simulink model "roachf_2048ch"  (Simulink 7.5)
settings: Solver=ode45  StartTime=0.0  StopTime=10.0  RelTol=1e-3
undefined symbols (not defined in the file or in its folder): Down, quant, ROACH, Up
libraries: xbsIndex_r4 x1405, xps_library x39, xbsReplacements_r4 x14, casper_library_misc x13, casper_library_delays x4, casper_library_sources x4, simulink x1
(part 6 of 14)

== system roachf_2048ch/WGNs/noise3 ==
  seed : Inport
  ld : Inport  Port=2
  Reinterpret : xbsIndex_r4/Reinterpret  force_arith_type=off  arith_type=Unsigned  force_bin_pt=on  bin_pt=7  block_type=reinterpret
      settings: infoedit="Changes signal type without altering the binary representation.   You can changed the signal between signed and unsigned, and relocate the binary point.<P><P>Hardware notes: In hardware this block costs nothing.<P><P>Example:  Suppose the input is 6 bits wide, signed, with 2 fractional bits, and the output is forced to unsigned with 0 fractional bits.  Then an input of -2.0 (1110.00 in binary 2's complement) becomes an output of 56 (111000 in binary)."  block_version=10.1.3
  Reinterpret1 : xbsIndex_r4/Reinterpret  force_arith_type=off  arith_type=Unsigned  force_bin_pt=on  bin_pt=7  block_type=reinterpret
      settings: infoedit="Changes signal type without altering the binary representation.   You can changed the signal between signed and unsigned, and relocate the binary point.<P><P>Hardware notes: In hardware this block costs nothing.<P><P>Example:  Suppose the input is 6 bits wide, signed, with 2 fractional bits, and the output is forced to unsigned with 0 fractional bits.  Then an input of -2.0 (1110.00 in binary 2's complement) becomes an output of 56 (111000 in binary)."  block_version=10.1.3
  Scale : xbsIndex_r4/Scale  scale_factor=4  dbl_ovrd=off  block_type=scale
      settings: infoedit=Scales input by a power of two by adjusting the binary point position.<P><P>Hardware notes: In hardware this block costs nothing.  block_version=10.1.3
  Scale1 : xbsIndex_r4/Scale  scale_factor=4  dbl_ovrd=off  block_type=scale
      settings: infoedit=Scales input by a power of two by adjusting the binary point position.<P><P>Hardware notes: In hardware this block costs nothing.  block_version=10.1.3
  convert : Subsystem  AncestorBlock=casper_library/Misc/convert  mask(convert){bin_pt_in=10, n_bits_out=8, bin_pt_out=0, quantization=Round  (unbiased: +/- Inf), overflow=Wrap, latency=1}
      mask prompts: bin_pt_in "Binary Point In"; n_bits_out "Bit Width Out"; bin_pt_out "Binary Point Out"
      mask help:
      | Convert input value to the specified bit width and precision.
      |
      | Does not support upscaling number of fractional bits (eg 8_5 to 8_4 is ok, but not 8_4 to 8_5).
      mask init: same as roachf_2048ch/WGNs/noise0/convert
      settings: AttributesFormatString=|
      | N_10 ==> 8_0
      | round inf, wrap
      | latency = 1
      mask Help:
      | <pre>
      | Description::
      | 
      | Outputs converted version of the input.
      | 
      | Mask Parameters::
      | 
      | Binary Point In (bin_pt_in): Specifies the binary point location in the input.
      | 
      | Bit Width Out (n_bits_out): Specifies the width of the output.
      | 
      | Binary Point Out (bin_pt_out): Specifies the binary point location in the output.
      | 
      | Quantization (quantization): Specifies quantization handling.
      | 
      | Overflow (overflow): Specifies overflow handling.
      | 
      | Latency (latency): Specifies the latency of the underlying adder block, which is the overall
      | latency of this block as well.
      | </pre>
      mask StyleString: edit,edit,edit,popup(Truncate|Round  (unbiased: +/- Inf)|Round  (unbiased: Even Values)|Round  (unbiased: Zero)|Round  (unbiased: Odd Values)|Round  (biased: Up)|Round  (biased: Down)),popup(Wrap|Saturate|Error),edit
  convert1 : Subsystem  AncestorBlock=casper_library/Misc/convert  mask(convert){bin_pt_in=10, n_bits_out=8, bin_pt_out=0, quantization=Round  (unbiased: +/- Inf), overflow=Wrap, latency=1}
      mask prompts: bin_pt_in "Binary Point In"; n_bits_out "Bit Width Out"; bin_pt_out "Binary Point Out"
      mask help:
      | Convert input value to the specified bit width and precision.
      |
      | Does not support upscaling number of fractional bits (eg 8_5 to 8_4 is ok, but not 8_4 to 8_5).
      mask init: same as roachf_2048ch/WGNs/noise0/convert
      settings: AttributesFormatString=|
      | N_10 ==> 8_0
      | round inf, wrap
      | latency = 1
      mask Help:
      | <pre>
      | Description::
      | 
      | Outputs converted version of the input.
      | 
      | Mask Parameters::
      | 
      | Binary Point In (bin_pt_in): Specifies the binary point location in the input.
      | 
      | Bit Width Out (n_bits_out): Specifies the width of the output.
      | 
      | Binary Point Out (bin_pt_out): Specifies the binary point location in the output.
      | 
      | Quantization (quantization): Specifies quantization handling.
      | 
      | Overflow (overflow): Specifies overflow handling.
      | 
      | Latency (latency): Specifies the latency of the underlying adder block, which is the overall
      | latency of this block as well.
      | </pre>
      mask StyleString: edit,edit,edit,popup(Truncate|Round  (unbiased: +/- Inf)|Round  (unbiased: Even Values)|Round  (unbiased: Zero)|Round  (unbiased: Odd Values)|Round  (biased: Up)|Round  (biased: Down)),popup(Wrap|Saturate|Error),edit
  wgn : Subsystem  AncestorBlock=casper_library_sources/White Gaussian Noise  mask(White Gaussian Noise Generator){seed=hex2dec('12345678')}
      mask help: Outputs two independent white gaussian noise signals as Fix_17_14 values with standard deviation 1.0, expected value 0.0, and crest factor 3.90625 (125/32).
      mask Help:
      | Initial seed is specified by a mask parameter at design time.  Can be reseeded at runtime by applying a UFix_32_0 value on the seed input and pulsing the load port (ld) high for one cycle.  Holding the load port high for more than one cycle is allowed, but it affects the underlying PRNG in undocumented ways.  Drill down into the subsystem if you want to learn more.
      | 
      | This block uses a TT800 uniform pseudo-random number generator followed by a uniform-to-normal converter implementing the Box-Muller Polar algorithm.
      | 
      | The TT800 is a high quality pseudo-random number generator based on a "twisted generialized linear feedback shift register".  Its output sequence repeats after 2^800 samples (~10^240 samples).  For more info see: Matsumoto, M. and Kurita, Y. 1994. "Twisted GFSR generators II", ACM Trans. Model. Comput. Simul. 4, 3 (Jul. 1994), 254-266 (http://doi.acm.org/10.1145/189443.189445).
      mask CallbackString:
      | if str2num(get_param(gcb, 'seed')) == 0
      |     error('Seed cannot be zero.')
      | end
      mask Display:
      | port_label('input',1,'seed');
      | port_label('input',2,'ld');
      | port_label('output',1,'n1');
      | port_label('output',2,'n2');
  n1 : Outport
  n2 : Outport  Port=2
  wires:
  wgn/1(n1) -> Scale/1
  wgn/2(n2) -> Scale1/1
  convert/1(out) -> Reinterpret/1
  convert1/1(out) -> Reinterpret1/1
  seed/1 -> wgn/1(seed)
  ld/1 -> wgn/2(ld)
  Scale/1 -> convert/1(in)
  Scale1/1 -> convert1/1(in)
  Reinterpret/1 -> n1/1
  Reinterpret1/1 -> n2/1

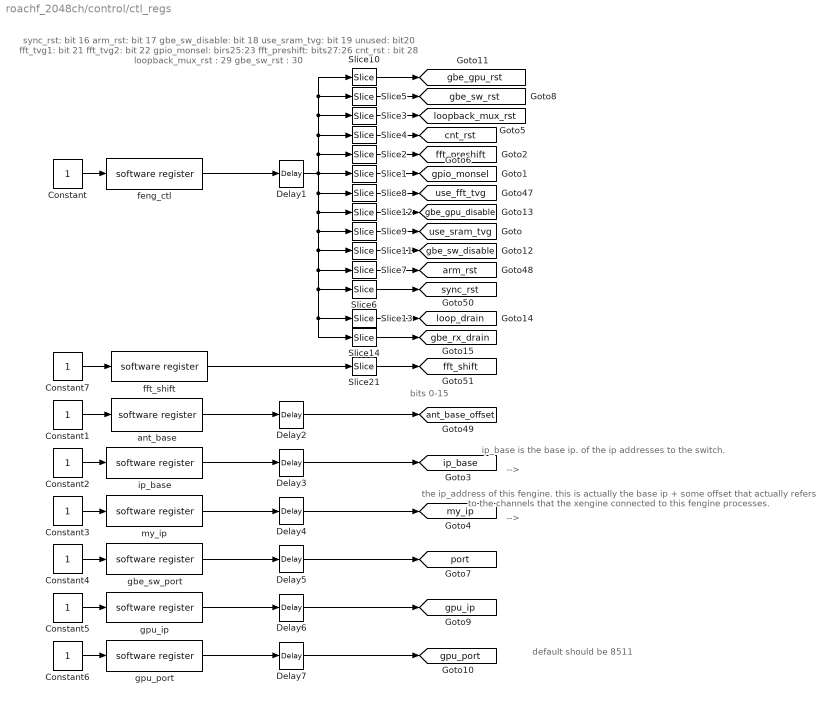
== system roachf_2048ch/control/ctl_regs ==
  note: sync_rst: bit 16
      | arm_rst: bit 17
      | gbe_sw_disable: bit 18
      | use_sram_tvg: bit 19
      | unused: bit20
      | fft_tvg1: bit 21
      | fft_tvg2: bit 22
      | gpio_monsel: birs25:23
      | fft_preshift: bits27:26
      | cnt_rst : bit 28
      | loopback_mux_rst : 29
      | gbe_sw_rst : 30
  note: ip_base is the base ip. of
      | the ip addresses to the switch.
  note: the ip_address of this fengine.
      | this is actually the base ip + some offset
      | that actually refers to the channels that
      | the xengine connected to this fengine
      | processes.
  note: -->
  note: -->
  note: default should be 8511
  note: bits 0-15
  Constant{,1..7} (8 alike) : Constant
  Delay{1..7} (7 alike) : xbsIndex_r4/Delay  rst=off  infoeditControl=Selection of Reset will increase slice count due to use of real FFs and instead of SRLs  en=off  latency=1  dbl_ovrd=off  reg_retiming=on  block_type=delay
      settings: xl_area=[0, 0, 0, 0, 0, 0, 0]
  Slice1 : xbsIndex_r4/Slice  nbits=3  boolean_output=off  mode=Lower Bit Location + Width  bit1=0  base1=MSB of Input  bit0=23  base0=LSB of Input  dbl_ovrd=off  block_type=slice
      settings: infoedit="Extracts a given range of bits from each input sample and presents it at the output.  The output type is ordinarily unsigned with binary point at zero, but can be Boolean when the slice is one bit wide.<P><P>Hardware notes: In hardware this block costs nothing."  block_version=10.1.3
  Slice10 : xbsIndex_r4/Slice  nbits=16  boolean_output=on  mode=Lower Bit Location + Width  bit1=0  base1=MSB of Input  bit0=31  base0=LSB of Input  dbl_ovrd=off  block_type=slice
      settings: block_version=10.1.3
  Slice11 : xbsIndex_r4/Slice  nbits=1  boolean_output=on  mode=Lower Bit Location + Width  bit1=0  base1=MSB of Input  bit0=18  base0=LSB of Input  dbl_ovrd=off  block_type=slice
      settings: block_version=10.1.3
  Slice12 : xbsIndex_r4/Slice  nbits=1  boolean_output=on  mode=Lower Bit Location + Width  bit1=0  base1=MSB of Input  bit0=20  base0=LSB of Input  dbl_ovrd=off  block_type=slice
      settings: block_version=10.1.3
  Slice13 : xbsIndex_r4/Slice  nbits=1  boolean_output=on  mode=Lower Bit Location + Width  bit1=0  base1=MSB of Input  bit0=0  base0=LSB of Input  dbl_ovrd=off  block_type=slice
      settings: block_version=10.1.3
  Slice14 : xbsIndex_r4/Slice  nbits=1  boolean_output=on  mode=Lower Bit Location + Width  bit1=0  base1=MSB of Input  bit0=1  base0=LSB of Input  dbl_ovrd=off  block_type=slice
      settings: block_version=10.1.3
  Slice2 : xbsIndex_r4/Slice  nbits=2  boolean_output=off  mode=Lower Bit Location + Width  bit1=0  base1=MSB of Input  bit0=26  base0=LSB of Input  dbl_ovrd=off  block_type=slice
      settings: infoedit="Extracts a given range of bits from each input sample and presents it at the output.  The output type is ordinarily unsigned with binary point at zero, but can be Boolean when the slice is one bit wide.<P><P>Hardware notes: In hardware this block costs nothing."  block_version=10.1.3
  Slice21 : xbsIndex_r4/Slice  nbits=16  boolean_output=off  mode=Lower Bit Location + Width  bit1=0  base1=MSB of Input  bit0=0  base0=LSB of Input  dbl_ovrd=off  block_type=slice
      settings: infoedit="Extracts a given range of bits from each input sample and presents it at the output.  The output type is ordinarily unsigned with binary point at zero, but can be Boolean when the slice is one bit wide.<P><P>Hardware notes: In hardware this block costs nothing."  block_version=10.1.3
  Slice3 : xbsIndex_r4/Slice  nbits=16  boolean_output=on  mode=Lower Bit Location + Width  bit1=0  base1=MSB of Input  bit0=29  base0=LSB of Input  dbl_ovrd=off  block_type=slice
      settings: block_version=10.1.3
  Slice4 : xbsIndex_r4/Slice  nbits=16  boolean_output=on  mode=Lower Bit Location + Width  bit1=0  base1=MSB of Input  bit0=28  base0=LSB of Input  dbl_ovrd=off  block_type=slice
      settings: block_version=10.1.3
  Slice5 : xbsIndex_r4/Slice  nbits=16  boolean_output=on  mode=Lower Bit Location + Width  bit1=0  base1=MSB of Input  bit0=30  base0=LSB of Input  dbl_ovrd=off  block_type=slice
      settings: block_version=10.1.3
  Slice6 : xbsIndex_r4/Slice  nbits=1  boolean_output=on  mode=Lower Bit Location + Width  bit1=0  base1=MSB of Input  bit0=16  base0=LSB of Input  dbl_ovrd=off  block_type=slice
      settings: infoedit="Extracts a given range of bits from each input sample and presents it at the output.  The output type is ordinarily unsigned with binary point at zero, but can be Boolean when the slice is one bit wide.<P><P>Hardware notes: In hardware this block costs nothing."  block_version=10.1.3
  Slice7 : xbsIndex_r4/Slice  nbits=1  boolean_output=on  mode=Lower Bit Location + Width  bit1=0  base1=MSB of Input  bit0=17  base0=LSB of Input  dbl_ovrd=off  block_type=slice
      settings: infoedit="Extracts a given range of bits from each input sample and presents it at the output.  The output type is ordinarily unsigned with binary point at zero, but can be Boolean when the slice is one bit wide.<P><P>Hardware notes: In hardware this block costs nothing."  block_version=10.1.3
  Slice8 : xbsIndex_r4/Slice  nbits=2  boolean_output=off  mode=Lower Bit Location + Width  bit1=0  base1=MSB of Input  bit0=21  base0=LSB of Input  dbl_ovrd=off  block_type=slice
      settings: infoedit="Extracts a given range of bits from each input sample and presents it at the output.  The output type is ordinarily unsigned with binary point at zero, but can be Boolean when the slice is one bit wide.<P><P>Hardware notes: In hardware this block costs nothing."  block_version=10.1.3
  Slice9 : xbsIndex_r4/Slice  nbits=1  boolean_output=off  mode=Lower Bit Location + Width  bit1=0  base1=MSB of Input  bit0=19  base0=LSB of Input  dbl_ovrd=off  block_type=slice
      settings: infoedit="Extracts a given range of bits from each input sample and presents it at the output.  The output type is ordinarily unsigned with binary point at zero, but can be Boolean when the slice is one bit wide.<P><P>Hardware notes: In hardware this block costs nothing."  block_version=10.1.3
  ant_base : xps_library/software register  Tag=xps:sw_reg  SystemSampleTime=-1  io_dir=From Processor  arith_type=Unsigned  bitwidth=32  bin_pt=0  sample_period=1  gw_name=roachf_2048ch_control_ctl_regs_ant_base_user_data_out
  feng_ctl : xps_library/software register  Tag=xps:sw_reg  SystemSampleTime=-1  io_dir=From Processor  arith_type=Unsigned  bitwidth=32  bin_pt=0  sample_period=1  gw_name=roachf_2048ch_control_ctl_regs_feng_ctl_user_data_out
  fft_shift : xps_library/software register  Tag=xps:sw_reg  SystemSampleTime=-1  io_dir=From Processor  arith_type=Unsigned  bitwidth=32  bin_pt=0  sample_period=1  gw_name=roachf_2048ch_control_ctl_regs_fft_shift_user_data_out
  gbe_sw_port : xps_library/software register  Tag=xps:sw_reg  SystemSampleTime=-1  io_dir=From Processor  arith_type=Unsigned  bitwidth=32  bin_pt=0  sample_period=1  gw_name=roachf_2048ch_control_ctl_regs_gbe_sw_port_user_data_out
  gpu_ip : xps_library/software register  Tag=xps:sw_reg  SystemSampleTime=-1  io_dir=From Processor  arith_type=Unsigned  bitwidth=32  bin_pt=0  sample_period=1  gw_name=roachf_2048ch_control_ctl_regs_gpu_ip_user_data_out
  gpu_port : xps_library/software register  Tag=xps:sw_reg  SystemSampleTime=-1  io_dir=From Processor  arith_type=Unsigned  bitwidth=32  bin_pt=0  sample_period=1  gw_name=roachf_2048ch_control_ctl_regs_gpu_port_user_data_out
  ip_base : xps_library/software register  Tag=xps:sw_reg  SystemSampleTime=-1  io_dir=From Processor  arith_type=Unsigned  bitwidth=32  bin_pt=0  sample_period=1  gw_name=roachf_2048ch_control_ctl_regs_ip_base_user_data_out
  my_ip : xps_library/software register  Tag=xps:sw_reg  SystemSampleTime=-1  io_dir=From Processor  arith_type=Unsigned  bitwidth=32  bin_pt=0  sample_period=1  gw_name=roachf_2048ch_control_ctl_regs_my_ip_user_data_out
  tag scope: ant_base_offset=global, arm_rst=global, cnt_rst=global, fft_preshift=global, fft_shift=global, gbe_gpu_disable=global, gbe_gpu_rst=global, gbe_rx_drain=global, gbe_sw_disable=global, gbe_sw_rst=global, gpio_monsel=global, gpu_ip=global, gpu_port=global, ip_base=global, loop_drain=global, loopback_mux_rst=global, my_ip=global, port=global, sync_rst=global, use_fft_tvg=global, use_sram_tvg=global
  wires:
  Delay2/1 -> [ant_base_offset]
  ant_base/1 -> Delay2/1
  Slice8/1 -> [use_fft_tvg]
  Delay1/1 -> Slice8/1, Slice7/1, Slice6/1, Slice14/1, Slice13/1, Slice11/1, Slice9/1, Slice12/1, Slice1/1, Slice2/1, Slice4/1, Slice3/1, Slice5/1, Slice10/1
  Slice21/1 -> [fft_shift]
  Slice6/1 -> [sync_rst]
  Slice7/1 -> [arm_rst]
  Slice9/1 -> [use_sram_tvg]
  Slice1/1 -> [gpio_monsel]
  Slice2/1 -> [fft_preshift]
  feng_ctl/1 -> Delay1/1
  Constant/1 -> feng_ctl/1
  Constant1/1 -> ant_base/1
  Constant2/1 -> ip_base/1
  Delay3/1 -> [ip_base]
  ip_base/1 -> Delay3/1
  Constant3/1 -> my_ip/1
  Delay4/1 -> [my_ip]
  my_ip/1 -> Delay4/1
  Slice4/1 -> [cnt_rst]
  Slice3/1 -> [loopback_mux_rst]
  Constant4/1 -> gbe_sw_port/1
  Delay5/1 -> [port]
  gbe_sw_port/1 -> Delay5/1
  Slice5/1 -> [gbe_sw_rst]
  Constant5/1 -> gpu_ip/1
  Delay6/1 -> [gpu_ip]
  gpu_ip/1 -> Delay6/1
  Constant6/1 -> gpu_port/1
  Delay7/1 -> [gpu_port]
  gpu_port/1 -> Delay7/1
  Slice10/1 -> [gbe_gpu_rst]
  Slice11/1 -> [gbe_sw_disable]
  Slice12/1 -> [gbe_gpu_disable]
  fft_shift/1 -> Slice21/1
  Constant7/1 -> fft_shift/1
  Slice13/1 -> [loop_drain]
  Slice14/1 -> [gbe_rx_drain]

== system roachf_2048ch/control/delay ==
  BitBasher : xbsIndex_r4/BitBasher  bitexpr=|  display_expr=off  sr_1=1  arith_type1=Unsigned  bin_pt1=0  sr_2=2  arith_type2=Unsigned  bin_pt2=0  sr_3=3  arith_type3=Unsigned  bin_pt3=0  sr_4=4  arith_type4=Unsigned  bin_pt4=0  dbl_ovrd=off  block_type=bitbasher
      | <html><head><meta name="qrichtext" content="1" /><style type="text/css">
      | p, li { white-space: pre-wrap; }
      | </style></head><body style=" font-family:'MS Shell Dlg 2'; font-size:8.25pt; font-weight:400; font-style:normal;">
      | <p style=" margin-top:12px; margin-bottom:12px; margin-left:0px; margin-right:0px; -qt-block-indent:0; text-indent:0px; font-family:'MS Shell Dlg'; font-size:8pt;">delay0={delay[3:0]}<br />delay1={delay[7:4]}<br />delay2={delay[11:8]}<br />delay3={delay[15:12]}</p></body></html>
      settings: block_version=10.1.3
  BitBasher1 : xbsIndex_r4/BitBasher  bitexpr=|  display_expr=off  sr_1=1  arith_type1=Unsigned  bin_pt1=0  sr_2=2  arith_type2=Unsigned  bin_pt2=0  sr_3=3  arith_type3=Unsigned  bin_pt3=0  sr_4=4  arith_type4=Unsigned  bin_pt4=0  dbl_ovrd=off  block_type=bitbasher
      | <html><head><meta name="qrichtext" content="1" /><style type="text/css">
      | p, li { white-space: pre-wrap; }
      | </style></head><body style=" font-family:'MS Shell Dlg 2'; font-size:8.25pt; font-weight:400; font-style:normal;">
      | <p style=" margin-top:12px; margin-bottom:12px; margin-left:0px; margin-right:0px; -qt-block-indent:0; text-indent:0px; font-family:'MS Shell Dlg'; font-size:8pt;">delay4={delay[19:16]}<br />delay5={delay[23:20]}<br />delay6={delay[27:24]}<br />delay7={delay[31:28]}</p></body></html>
      settings: block_version=10.1.3
  delay : xps_library/software register  Tag=xps:sw_reg  SystemSampleTime=-1  io_dir=From Processor  arith_type=Unsigned  bitwidth=32  bin_pt=0  sample_period=1  gw_name=roachf_2048ch_control_delay_delay_user_data_out
  tag scope: delay0=global, delay1=global, delay2=global, delay3=global, delay4=global, delay5=global, delay6=global, delay7=global
  wires:
  BitBasher/1 -> [delay0]
  BitBasher/2 -> [delay1]
  BitBasher/3 -> [delay2]
  BitBasher/4 -> [delay3]
  BitBasher1/1 -> [delay4]
  BitBasher1/2 -> [delay5]
  BitBasher1/3 -> [delay6]
  BitBasher1/4 -> [delay7]
  delay/1 -> BitBasher/1, BitBasher1/1

== system roachf_2048ch/control/eq_coefs ==
  Slice{1,6,9,22} (4 alike) : xbsIndex_r4/Slice  nbits=18  boolean_output=off  mode=Lower Bit Location + Width  bit1=0  base1=MSB of Input  bit0=0  base0=LSB of Input  dbl_ovrd=off  block_type=slice
      settings: infoedit="Extracts a given range of bits from each input sample and presents it at the output.  The output type is ordinarily unsigned with binary point at zero, but can be Boolean when the slice is one bit wide.<P><P>Hardware notes: In hardware this block costs nothing."  block_version=10.1.3
  Slice{2,4,7,10} (4 alike) : xbsIndex_r4/Slice  nbits=8  boolean_output=off  mode=Lower Bit Location + Width  bit1=0  base1=MSB of Input  bit0=18  base0=LSB of Input  dbl_ovrd=off  block_type=slice
      settings: block_version=10.1.3
  Slice{3,5,8,11} (4 alike) : xbsIndex_r4/Slice  nbits=18  boolean_output=on  mode=Upper Bit Location + Width  bit1=0  base1=MSB of Input  bit0=0  base0=LSB of Input  dbl_ovrd=off  block_type=slice
      settings: block_version=10.1.3
  eq0_ctl : xps_library/software register  Tag=xps:sw_reg  SystemSampleTime=-1  io_dir=From Processor  arith_type=Unsigned  bitwidth=32  bin_pt=0  sample_period=1  gw_name=roachf_2048ch_control_eq_coefs_eq0_ctl_user_data_out
  eq1_ctl : xps_library/software register  Tag=xps:sw_reg  SystemSampleTime=-1  io_dir=From Processor  arith_type=Unsigned  bitwidth=32  bin_pt=0  sample_period=1  gw_name=roachf_2048ch_control_eq_coefs_eq1_ctl_user_data_out
  eq2_ctl : xps_library/software register  Tag=xps:sw_reg  SystemSampleTime=-1  io_dir=From Processor  arith_type=Unsigned  bitwidth=32  bin_pt=0  sample_period=1  gw_name=roachf_2048ch_control_eq_coefs_eq2_ctl_user_data_out
  eq3_ctl : xps_library/software register  Tag=xps:sw_reg  SystemSampleTime=-1  io_dir=From Processor  arith_type=Unsigned  bitwidth=32  bin_pt=0  sample_period=1  gw_name=roachf_2048ch_control_eq_coefs_eq3_ctl_user_data_out
  eq_coeff0 : Subsystem  mask{addr_width=6, addr_offset=0}
      mask prompts: addr_width "Number of addresses (2^?)"; addr_offset "Address block offset (multiple of above)"
      mask init:
      | start_addr = 2^addr_width*(addr_offset);
      | end_addr = start_addr + 2^addr_width - 1;
      | fmtstr = sprintf('Mapped address range: %d-%d', start_addr,end_addr);
      | set_param(gcb, 'AttributesFormatString', fmtstr);
      settings: AttributesFormatString=Mapped address range: 0-63
  eq_coeff1 : Subsystem  mask{addr_width=6, addr_offset=1}
      mask prompts: addr_width "Number of addresses (2^?)"; addr_offset "Address block offset (multiple of above)"
      mask init: same as roachf_2048ch/control/eq_coefs/eq_coeff0
      settings: AttributesFormatString=Mapped address range: 64-127
  eq_coeff2 : Subsystem  mask{addr_width=6, addr_offset=2}
      mask prompts: addr_width "Number of addresses (2^?)"; addr_offset "Address block offset (multiple of above)"
      mask init: same as roachf_2048ch/control/eq_coefs/eq_coeff0
      settings: AttributesFormatString=Mapped address range: 128-191
  eq_coeff3 : Subsystem  mask{addr_width=6, addr_offset=3}
      mask prompts: addr_width "Number of addresses (2^?)"; addr_offset "Address block offset (multiple of above)"
      mask init: same as roachf_2048ch/control/eq_coefs/eq_coeff0
      settings: AttributesFormatString=Mapped address range: 192-255
  tag scope: eq_addr_0=global, eq_addr_1=global, eq_addr_2=global, eq_addr_3=global, eq_data_0=global, eq_data_1=global, eq_data_2=global, eq_data_3=global, eq_en_0=global, eq_en_1=global, eq_en_2=global, eq_en_3=global
  wires:
  eq_coeff1/1(data_out) -> [eq_data_1]
  eq_coeff1/2(addr_out) -> [eq_addr_1]
  eq_coeff1/3(valid_out) -> [eq_en_1]
  eq_coeff2/1(data_out) -> [eq_data_2]
  eq_coeff2/2(addr_out) -> [eq_addr_2]
  eq_coeff2/3(valid_out) -> [eq_en_2]
  Slice1/1 -> eq_coeff1/1(data_in)
  Slice6/1 -> eq_coeff2/1(data_in)
  eq_coeff3/1(data_out) -> [eq_data_3]
  eq_coeff3/2(addr_out) -> [eq_addr_3]
  eq_coeff3/3(valid_out) -> [eq_en_3]
  Slice9/1 -> eq_coeff3/1(data_in)
  eq_coeff0/1(data_out) -> [eq_data_0]
  eq_coeff0/2(addr_out) -> [eq_addr_0]
  eq_coeff0/3(valid_out) -> [eq_en_0]
  Slice22/1 -> eq_coeff0/1(data_in)
  eq0_ctl/1 -> Slice22/1, Slice4/1, Slice5/1
  Slice4/1 -> eq_coeff0/2(addr_in)
  Slice5/1 -> eq_coeff0/3(valid_in)
  eq1_ctl/1 -> Slice1/1, Slice2/1, Slice3/1
  Slice2/1 -> eq_coeff1/2(addr_in)
  Slice3/1 -> eq_coeff1/3(valid_in)
  eq2_ctl/1 -> Slice6/1, Slice7/1, Slice8/1
  Slice7/1 -> eq_coeff2/2(addr_in)
  Slice8/1 -> eq_coeff2/3(valid_in)
  eq3_ctl/1 -> Slice9/1, Slice10/1, Slice11/1
  Slice10/1 -> eq_coeff3/2(addr_in)
  Slice11/1 -> eq_coeff3/3(valid_in)

== system roachf_2048ch/control/insel ==
  BitBasher : xbsIndex_r4/BitBasher  bitexpr=|  display_expr=off  sr_1=1  arith_type1=Unsigned  bin_pt1=0  sr_2=2  arith_type2=Unsigned  bin_pt2=0  sr_3=3  arith_type3=Unsigned  bin_pt3=0  sr_4=4  arith_type4=Unsigned  bin_pt4=0  dbl_ovrd=off  block_type=bitbasher
      | <html><head><meta name="qrichtext" content="1" /><style type="text/css">
      | p, li { white-space: pre-wrap; }
      | </style></head><body style=" font-family:'MS Shell Dlg 2'; font-size:8.25pt; font-weight:400; font-style:normal;">
      | <p style=" margin-top:12px; margin-bottom:12px; margin-left:0px; margin-right:0px; -qt-block-indent:0; text-indent:0px; font-family:'MS Shell Dlg'; font-size:8pt;">insel0={insel[1:0]}<br />insel1={insel[5:4]}<br />insel2={insel[9:8]}<br />insel3={insel[13:12]}</p></body></html>
      settings: block_version=10.1.3
  BitBasher1 : xbsIndex_r4/BitBasher  bitexpr=|  display_expr=off  sr_1=1  arith_type1=Unsigned  bin_pt1=0  sr_2=2  arith_type2=Unsigned  bin_pt2=0  sr_3=3  arith_type3=Unsigned  bin_pt3=0  sr_4=4  arith_type4=Unsigned  bin_pt4=0  dbl_ovrd=off  block_type=bitbasher
      | <html><head><meta name="qrichtext" content="1" /><style type="text/css">
      | p, li { white-space: pre-wrap; }
      | </style></head><body style=" font-family:'MS Shell Dlg 2'; font-size:8.25pt; font-weight:400; font-style:normal;">
      | <p style=" margin-top:12px; margin-bottom:12px; margin-left:0px; margin-right:0px; -qt-block-indent:0; text-indent:0px; font-family:'MS Shell Dlg'; font-size:8pt;">insel4={insel[17:16]}<br />insel5={insel[21:20]}<br />insel6={insel[25:24]}<br />insel7={insel[29:28]}</p></body></html>
      settings: block_version=10.1.3
  insel : xps_library/software register  Tag=xps:sw_reg  SystemSampleTime=-1  io_dir=From Processor  arith_type=Unsigned  bitwidth=32  bin_pt=0  sample_period=1  gw_name=roachf_2048ch_control_insel_insel_user_data_out
  tag scope: insel0=global, insel1=global, insel2=global, insel3=global, insel4=global, insel5=global, insel6=global, insel7=global
  wires:
  BitBasher/1 -> [insel0]
  BitBasher/2 -> [insel1]
  BitBasher/3 -> [insel2]
  BitBasher/4 -> [insel3]
  BitBasher1/1 -> [insel4]
  BitBasher1/2 -> [insel5]
  BitBasher1/3 -> [insel6]
  BitBasher1/4 -> [insel7]
  insel/1 -> BitBasher/1, BitBasher1/1

== system roachf_2048ch/control/seed ==
  BitBasher : xbsIndex_r4/BitBasher  bitexpr=|  display_expr=off  sr_1=1  arith_type1=Unsigned  bin_pt1=0  sr_2=2  arith_type2=Unsigned  bin_pt2=0  sr_3=3  arith_type3=Unsigned  bin_pt3=0  sr_4=4  arith_type4=Unsigned  bin_pt4=0  dbl_ovrd=off  block_type=bitbasher
      | <html><head><meta name="qrichtext" content="1" /><style type="text/css">
      | p, li { white-space: pre-wrap; }
      | </style></head><body style=" font-family:'MS Shell Dlg 2'; font-size:8.25pt; font-weight:400; font-style:normal;">
      | <p style=" margin-top:12px; margin-bottom:12px; margin-left:0px; margin-right:0px; -qt-block-indent:0; text-indent:0px; font-family:'MS Shell Dlg'; font-size:8pt;">seed0={8'h5c, seed[7:0], seed[0:7], 8'ha3}<br />seed1={8'h5c, seed[15:8], seed[8:15], 8'ha3}<br />seed2={8'h5c, seed[23:16], seed[16:23], 8'ha3}<br />seed3={8'h5c, seed[31:24], seed[24:31], 8'ha3}</p></body></html>
      settings: block_version=10.1.3
  armed_trigger : casper_library_misc/armed_trigger  SystemSampleTime=-1  hidden=0
  seed_data : xps_library/software register  Tag=xps:sw_reg  SystemSampleTime=-1  io_dir=From Processor  arith_type=Unsigned  bitwidth=32  bin_pt=0  sample_period=1  gw_name=roachf_2048ch_control_seed_seed_data_user_data_out
  tag scope: seed0=global, seed1=global, seed2=global, seed3=global, seed_ld=global
  wires:
  BitBasher/1 -> [seed0]
  BitBasher/2 -> [seed1]
  BitBasher/3 -> [seed2]
  BitBasher/4 -> [seed3]
  armed_trigger/1 -> [seed_ld]
  [sync_gen] -> armed_trigger/2
  seed_data/1 -> BitBasher/1
  [arm_rst] -> armed_trigger/1

== system roachf_2048ch/input_mux/muxin0 ==
  sel : Inport
  adc : Inport  Port=2
  n0 : Inport  Port=3
  n1 : Inport  Port=4
  delay : Inport  Port=5
  Addressable Shift Register : xbsIndex_r4/Addressable Shift Register  infer_latency=on  depth=2  initVector=[0]  en=off  dbl_ovrd=off  use_behavioral_HDL=off  Optimization=Resource  use_rpm=off  block_type=addrsr
      settings: infoedit="Delay of configurable length.  Any element in the delay line can be addressed and driven onto the output port.<br><br>Hardware notes: Implemented using SRL16s.  If Virtex-4, Virtex-II or Spartan-3 devices are used, multiple SRLC16s are cascaded together."  block_version=10.1.3
  Constant : xbsIndex_r4/Constant  const=0  gui_display_data_type=Fixed-point  arith_type=Signed (2's comp)  n_bits=8  bin_pt=7  preci_type=Single  exp_width=8  frac_width=24  explicit_period=on  period=1  equ=P=C  opselect=C  inp2=PCIN>>17  opr=+  inp1=P  carry=CIN  dbl_ovrd=off  block_type=constant
  Mux : xbsIndex_r4/Mux  inputs=4  en=off  latency=1  precision=Full  arith_type=Unsigned  n_bits=16  bin_pt=14  quantization=Truncate  overflow=Wrap  dbl_ovrd=off  block_type=mux
  out : Outport
  wires:
  Mux/1 -> Addressable Shift Register/1
  sel/1 -> Mux/1
  adc/1 -> Mux/2
  n0/1 -> Mux/3
  Addressable Shift Register/1 -> out/1
  n1/1 -> Mux/4
  delay/1 -> Addressable Shift Register/2
  Constant/1 -> Mux/5

== system roachf_2048ch/input_mux/muxin1 ==
  sel : Inport
  adc : Inport  Port=2
  n0 : Inport  Port=3
  n1 : Inport  Port=4
  delay : Inport  Port=5
  Addressable Shift Register : xbsIndex_r4/Addressable Shift Register  infer_latency=on  depth=2  initVector=[0]  en=off  dbl_ovrd=off  use_behavioral_HDL=off  Optimization=Resource  use_rpm=off  block_type=addrsr
      settings: infoedit="Delay of configurable length.  Any element in the delay line can be addressed and driven onto the output port.<br><br>Hardware notes: Implemented using SRL16s.  If Virtex-4, Virtex-II or Spartan-3 devices are used, multiple SRLC16s are cascaded together."  block_version=10.1.3
  Constant : xbsIndex_r4/Constant  const=0  gui_display_data_type=Fixed-point  arith_type=Signed (2's comp)  n_bits=8  bin_pt=7  preci_type=Single  exp_width=8  frac_width=24  explicit_period=on  period=1  equ=P=C  opselect=C  inp2=PCIN>>17  opr=+  inp1=P  carry=CIN  dbl_ovrd=off  block_type=constant
  Mux : xbsIndex_r4/Mux  inputs=4  en=off  latency=1  precision=Full  arith_type=Unsigned  n_bits=16  bin_pt=14  quantization=Truncate  overflow=Wrap  dbl_ovrd=off  block_type=mux
  out : Outport
  wires:
  Mux/1 -> Addressable Shift Register/1
  sel/1 -> Mux/1
  adc/1 -> Mux/2
  n0/1 -> Mux/3
  Addressable Shift Register/1 -> out/1
  n1/1 -> Mux/4
  delay/1 -> Addressable Shift Register/2
  Constant/1 -> Mux/5

== system roachf_2048ch/input_mux/muxin2 ==
  sel : Inport
  adc : Inport  Port=2
  n0 : Inport  Port=3
  n1 : Inport  Port=4
  delay : Inport  Port=5
  Addressable Shift Register : xbsIndex_r4/Addressable Shift Register  infer_latency=on  depth=2  initVector=[0]  en=off  dbl_ovrd=off  use_behavioral_HDL=off  Optimization=Resource  use_rpm=off  block_type=addrsr
      settings: infoedit="Delay of configurable length.  Any element in the delay line can be addressed and driven onto the output port.<br><br>Hardware notes: Implemented using SRL16s.  If Virtex-4, Virtex-II or Spartan-3 devices are used, multiple SRLC16s are cascaded together."  block_version=10.1.3
  Constant : xbsIndex_r4/Constant  const=0  gui_display_data_type=Fixed-point  arith_type=Signed (2's comp)  n_bits=8  bin_pt=7  preci_type=Single  exp_width=8  frac_width=24  explicit_period=on  period=1  equ=P=C  opselect=C  inp2=PCIN>>17  opr=+  inp1=P  carry=CIN  dbl_ovrd=off  block_type=constant
  Mux : xbsIndex_r4/Mux  inputs=4  en=off  latency=1  precision=Full  arith_type=Unsigned  n_bits=16  bin_pt=14  quantization=Truncate  overflow=Wrap  dbl_ovrd=off  block_type=mux
  out : Outport
  wires:
  Mux/1 -> Addressable Shift Register/1
  sel/1 -> Mux/1
  adc/1 -> Mux/2
  n0/1 -> Mux/3
  Addressable Shift Register/1 -> out/1
  n1/1 -> Mux/4
  delay/1 -> Addressable Shift Register/2
  Constant/1 -> Mux/5

== system roachf_2048ch/input_mux/muxin3 ==
  sel : Inport
  adc : Inport  Port=2
  n0 : Inport  Port=3
  n1 : Inport  Port=4
  delay : Inport  Port=5
  Addressable Shift Register : xbsIndex_r4/Addressable Shift Register  infer_latency=on  depth=2  initVector=[0]  en=off  dbl_ovrd=off  use_behavioral_HDL=off  Optimization=Resource  use_rpm=off  block_type=addrsr
      settings: infoedit="Delay of configurable length.  Any element in the delay line can be addressed and driven onto the output port.<br><br>Hardware notes: Implemented using SRL16s.  If Virtex-4, Virtex-II or Spartan-3 devices are used, multiple SRLC16s are cascaded together."  block_version=10.1.3
  Constant : xbsIndex_r4/Constant  const=0  gui_display_data_type=Fixed-point  arith_type=Signed (2's comp)  n_bits=8  bin_pt=7  preci_type=Single  exp_width=8  frac_width=24  explicit_period=on  period=1  equ=P=C  opselect=C  inp2=PCIN>>17  opr=+  inp1=P  carry=CIN  dbl_ovrd=off  block_type=constant
  Mux : xbsIndex_r4/Mux  inputs=4  en=off  latency=1  precision=Full  arith_type=Unsigned  n_bits=16  bin_pt=14  quantization=Truncate  overflow=Wrap  dbl_ovrd=off  block_type=mux
  out : Outport
  wires:
  Mux/1 -> Addressable Shift Register/1
  sel/1 -> Mux/1
  adc/1 -> Mux/2
  n0/1 -> Mux/3
  Addressable Shift Register/1 -> out/1
  n1/1 -> Mux/4
  delay/1 -> Addressable Shift Register/2
  Constant/1 -> Mux/5

== system roachf_2048ch/input_mux/muxin4 ==
  sel : Inport
  adc : Inport  Port=2
  n0 : Inport  Port=3
  n1 : Inport  Port=4
  delay : Inport  Port=5
  Addressable Shift Register : xbsIndex_r4/Addressable Shift Register  infer_latency=on  depth=2  initVector=[0]  en=off  dbl_ovrd=off  use_behavioral_HDL=off  Optimization=Resource  use_rpm=off  block_type=addrsr
      settings: infoedit="Delay of configurable length.  Any element in the delay line can be addressed and driven onto the output port.<br><br>Hardware notes: Implemented using SRL16s.  If Virtex-4, Virtex-II or Spartan-3 devices are used, multiple SRLC16s are cascaded together."  block_version=10.1.3
  Constant : xbsIndex_r4/Constant  const=0  gui_display_data_type=Fixed-point  arith_type=Signed (2's comp)  n_bits=8  bin_pt=7  preci_type=Single  exp_width=8  frac_width=24  explicit_period=on  period=1  equ=P=C  opselect=C  inp2=PCIN>>17  opr=+  inp1=P  carry=CIN  dbl_ovrd=off  block_type=constant
  Mux : xbsIndex_r4/Mux  inputs=4  en=off  latency=1  precision=Full  arith_type=Unsigned  n_bits=16  bin_pt=14  quantization=Truncate  overflow=Wrap  dbl_ovrd=off  block_type=mux
  out : Outport
  wires:
  Mux/1 -> Addressable Shift Register/1
  sel/1 -> Mux/1
  adc/1 -> Mux/2
  n0/1 -> Mux/3
  Addressable Shift Register/1 -> out/1
  n1/1 -> Mux/4
  delay/1 -> Addressable Shift Register/2
  Constant/1 -> Mux/5

== system roachf_2048ch/input_mux/muxin5 ==
  sel : Inport
  adc : Inport  Port=2
  n0 : Inport  Port=3
  n1 : Inport  Port=4
  delay : Inport  Port=5
  Addressable Shift Register : xbsIndex_r4/Addressable Shift Register  infer_latency=on  depth=2  initVector=[0]  en=off  dbl_ovrd=off  use_behavioral_HDL=off  Optimization=Resource  use_rpm=off  block_type=addrsr
      settings: infoedit="Delay of configurable length.  Any element in the delay line can be addressed and driven onto the output port.<br><br>Hardware notes: Implemented using SRL16s.  If Virtex-4, Virtex-II or Spartan-3 devices are used, multiple SRLC16s are cascaded together."  block_version=10.1.3
  Constant : xbsIndex_r4/Constant  const=0  gui_display_data_type=Fixed-point  arith_type=Signed (2's comp)  n_bits=8  bin_pt=7  preci_type=Single  exp_width=8  frac_width=24  explicit_period=on  period=1  equ=P=C  opselect=C  inp2=PCIN>>17  opr=+  inp1=P  carry=CIN  dbl_ovrd=off  block_type=constant
  Mux : xbsIndex_r4/Mux  inputs=4  en=off  latency=1  precision=Full  arith_type=Unsigned  n_bits=16  bin_pt=14  quantization=Truncate  overflow=Wrap  dbl_ovrd=off  block_type=mux
  out : Outport
  wires:
  Mux/1 -> Addressable Shift Register/1
  sel/1 -> Mux/1
  adc/1 -> Mux/2
  n0/1 -> Mux/3
  Addressable Shift Register/1 -> out/1
  n1/1 -> Mux/4
  delay/1 -> Addressable Shift Register/2
  Constant/1 -> Mux/5

== system roachf_2048ch/input_mux/muxin6 ==
  sel : Inport
  adc : Inport  Port=2
  n0 : Inport  Port=3
  n1 : Inport  Port=4
  delay : Inport  Port=5
  Addressable Shift Register : xbsIndex_r4/Addressable Shift Register  infer_latency=on  depth=2  initVector=[0]  en=off  dbl_ovrd=off  use_behavioral_HDL=off  Optimization=Resource  use_rpm=off  block_type=addrsr
      settings: infoedit="Delay of configurable length.  Any element in the delay line can be addressed and driven onto the output port.<br><br>Hardware notes: Implemented using SRL16s.  If Virtex-4, Virtex-II or Spartan-3 devices are used, multiple SRLC16s are cascaded together."  block_version=10.1.3
  Constant : xbsIndex_r4/Constant  const=0  gui_display_data_type=Fixed-point  arith_type=Signed (2's comp)  n_bits=8  bin_pt=7  preci_type=Single  exp_width=8  frac_width=24  explicit_period=on  period=1  equ=P=C  opselect=C  inp2=PCIN>>17  opr=+  inp1=P  carry=CIN  dbl_ovrd=off  block_type=constant
  Mux : xbsIndex_r4/Mux  inputs=4  en=off  latency=1  precision=Full  arith_type=Unsigned  n_bits=16  bin_pt=14  quantization=Truncate  overflow=Wrap  dbl_ovrd=off  block_type=mux
  out : Outport
  wires:
  Mux/1 -> Addressable Shift Register/1
  sel/1 -> Mux/1
  adc/1 -> Mux/2
  n0/1 -> Mux/3
  Addressable Shift Register/1 -> out/1
  n1/1 -> Mux/4
  delay/1 -> Addressable Shift Register/2
  Constant/1 -> Mux/5

== system roachf_2048ch/input_mux/muxin7 ==
  sel : Inport
  adc : Inport  Port=2
  n0 : Inport  Port=3
  n1 : Inport  Port=4
  delay : Inport  Port=5
  Addressable Shift Register : xbsIndex_r4/Addressable Shift Register  infer_latency=on  depth=2  initVector=[0]  en=off  dbl_ovrd=off  use_behavioral_HDL=off  Optimization=Resource  use_rpm=off  block_type=addrsr
      settings: infoedit="Delay of configurable length.  Any element in the delay line can be addressed and driven onto the output port.<br><br>Hardware notes: Implemented using SRL16s.  If Virtex-4, Virtex-II or Spartan-3 devices are used, multiple SRLC16s are cascaded together."  block_version=10.1.3
  Constant : xbsIndex_r4/Constant  const=0  gui_display_data_type=Fixed-point  arith_type=Signed (2's comp)  n_bits=8  bin_pt=7  preci_type=Single  exp_width=8  frac_width=24  explicit_period=on  period=1  equ=P=C  opselect=C  inp2=PCIN>>17  opr=+  inp1=P  carry=CIN  dbl_ovrd=off  block_type=constant
  Mux : xbsIndex_r4/Mux  inputs=4  en=off  latency=1  precision=Full  arith_type=Unsigned  n_bits=16  bin_pt=14  quantization=Truncate  overflow=Wrap  dbl_ovrd=off  block_type=mux
  out : Outport
  wires:
  Mux/1 -> Addressable Shift Register/1
  sel/1 -> Mux/1
  adc/1 -> Mux/2
  n0/1 -> Mux/3
  Addressable Shift Register/1 -> out/1
  n1/1 -> Mux/4
  delay/1 -> Addressable Shift Register/2
  Constant/1 -> Mux/5

== system roachf_2048ch/2GPU/10gbetxsnap/bram_lsb ==
  addr : Inport
  data_in : Inport  Port=2
  we : Inport  Port=3
  calc_add : Subsystem
  convert_addr : xbsIndex_r4/Convert  gui_display_data_type=Fixed-point  arith_type=Unsigned  n_bits=addr_width  bin_pt=0  float_type=Single  exp_bits=8  fraction_bits=24  quantization=Truncate  overflow=Wrap  en=off  latency=0  dbl_ovrd=off  pipeline=off  block_type=convert
      settings: xl_area=[0, 0, 0, 0, 0, 0, 0]
  convert_din : xbsIndex_r4/Convert  gui_display_data_type=Fixed-point  arith_type=Unsigned  n_bits=data_width  bin_pt=data_bin_pt  float_type=Single  exp_bits=8  fraction_bits=24  quantization=Truncate  overflow=Wrap  en=off  latency=0  dbl_ovrd=off  pipeline=off  block_type=convert
      settings: xl_area=[0, 0, 0, 0, 0, 0, 0]
  convert_din1 : xbsIndex_r4/Convert  gui_display_data_type=Fixed-point  arith_type=Unsigned  n_bits=data_width  bin_pt=data_bin_pt  float_type=Single  exp_bits=8  fraction_bits=24  quantization=Truncate  overflow=Wrap  en=off  latency=0  dbl_ovrd=off  pipeline=off  block_type=convert
      settings: xl_area=[0, 0, 0, 0, 0, 0, 0]
  convert_we : xbsIndex_r4/Convert  gui_display_data_type=Fixed-point  arith_type=Unsigned  n_bits=1  bin_pt=0  float_type=Single  exp_bits=8  fraction_bits=24  quantization=Truncate  overflow=Wrap  en=off  latency=0  dbl_ovrd=off  pipeline=off  block_type=convert
      settings: xl_area=[0, 0, 0, 0, 0, 0, 0]
  mem : Subsystem
  munge_in : Subsystem  AncestorBlock=casper_library_flow_control/munge  mask(munge){divisions=1, div_size=32, order=[0]}
      mask prompts: divisions "Number of divisions"; div_size "Division size (bits)"; order "Division packing order"
      mask help: Splits an input bus into the specified number of divisions and then recombines them in the order specified (most significant division = 0,least = number divisions-1)
      mask init:
      | munge_init(gcb, ...
      |     'divisions', divisions, ...
      |     'div_size', div_size, ...
      |     'order', order);
      settings: AttributesFormatString=|
      | [0]
      | 32 bits
  munge_out : Subsystem  AncestorBlock=casper_library_flow_control/munge  mask(munge){divisions=1, div_size=32, order=[0]}
      mask prompts: divisions "Number of divisions"; div_size "Division size (bits)"; order "Division packing order"
      mask help: Splits an input bus into the specified number of divisions and then recombines them in the order specified (most significant division = 0,least = number divisions-1)
      mask init:
      | munge_init(gcb, ...
      |     'divisions', divisions, ...
      |     'div_size', div_size, ...
      |     'order', order);
      settings: AttributesFormatString=|
      | [0]
      | 32 bits
  roachf_2048ch_2GPU_10gbetxsnap_bram_lsb_addr : xbsIndex_r4/Gateway Out  hdl_port=on  timing_constraint=None  locs_specified=off  LOCs={'A5','B9','A9','C1','A3','G6','E9','A6','A7','A8','B8','B1','B3','D9','B5','B4','B6','C2'}  block_type=gatewayout
      settings: infoedit="Gateway out block.  Converts Xilinx fixed point inputs into ouputs of type Simulink integer, double, or fixed point.<P><P>Hardware notes:  In hardware these blocks become top level output ports or are discarded, depending on how they are configured."  xl_area=[0, 0, 0, 0, 0, 0, 0]  sginterface={'Nallatech'=>{'xdspkit'=>{'non_memory_mapped_port'=>'uprev_Shared_BRAM_addr'}},'Xilinx'=>{'jtaghwcosim'=>{'non_memory_mapped_port'=>'uprev_Shared_BRAM_addr'},'xdspkit'=>{'non_memory_mapped_port'=>'uprev_Shared_BRAM_addr'}}}
  roachf_2048ch_2GPU_10gbetxsnap_bram_lsb_data_in : xbsIndex_r4/Gateway Out  hdl_port=on  timing_constraint=None  locs_specified=off  LOCs={'B21','B22','A22','B23','B19','C19','A20','A21','A23','B24','A24','A25','E18','D18','C18','B18'}  block_type=gatewayout
      settings: infoedit="Gateway out block.  Converts Xilinx fixed point inputs into ouputs of type Simulink integer, double, or fixed point.<P><P>Hardware notes:  In hardware these blocks become top level output ports or are discarded, depending on how they are configured."  xl_area=[0, 0, 0, 0, 0, 0, 0]  sginterface={'Nallatech'=>{'xdspkit'=>{'non_memory_mapped_port'=>'uprev_Shared_BRAM_data_in'}},'Xilinx'=>{'jtaghwcosim'=>{'non_memory_mapped_port'=>'uprev_Shared_BRAM_data_in'},'xdspkit'=>{'non_memory_mapped_port'=>'uprev_Shared_BRAM_data_in'}}}
  roachf_2048ch_2GPU_10gbetxsnap_bram_lsb_data_out : xbsIndex_r4/Gateway In  gui_display_data_type=Fixed-point  arith_type=Unsigned  n_bits=data_width  bin_pt=data_bin_pt  preci_type=Single  exp_width=8  frac_width=24  quantization=Truncate  overflow=Wrap  period=sample_rate  dbl_ovrd=off  timing_constraint=None  locs_specified=off  LOCs={}  hdl_port=on  block_type=gatewayin
      settings: infoedit="Gateway in block.  Converts inputs of type Simulink integer, double and fixed point to  Xilinx fixed point type.<br><br>Hardware notes:  In hardware these blocks become top level input ports."  xl_area=[0, 0, 0, 0, 0, 0, 0]
  roachf_2048ch_2GPU_10gbetxsnap_bram_lsb_we : xbsIndex_r4/Gateway Out  hdl_port=on  timing_constraint=None  locs_specified=off  LOCs={'A14'}  block_type=gatewayout
      settings: infoedit="Gateway out block.  Converts Xilinx fixed point inputs into ouputs of type Simulink integer, double, or fixed point.<P><P>Hardware notes:  In hardware these blocks become top level output ports or are discarded, depending on how they are configured."  xl_area=[0, 0, 0, 0, 0, 0, 0]
  data_out : Outport
  wires:
  mem/1(Out1) -> roachf_2048ch_2GPU_10gbetxsnap_bram_lsb_data_out/1
  data_in/1 -> convert_din/1
  roachf_2048ch_2GPU_10gbetxsnap_bram_lsb_data_out/1 -> munge_out/1(din)
  addr/1 -> calc_add/1(in)
  we/1 -> convert_we/1
  convert_we/1 -> roachf_2048ch_2GPU_10gbetxsnap_bram_lsb_we/1
  roachf_2048ch_2GPU_10gbetxsnap_bram_lsb_addr/1 -> mem/1(In1)
  roachf_2048ch_2GPU_10gbetxsnap_bram_lsb_data_in/1 -> mem/2(In2)
  roachf_2048ch_2GPU_10gbetxsnap_bram_lsb_we/1 -> mem/3(In3)
  munge_in/1(dout) -> convert_din1/1
  munge_out/1(dout) -> data_out/1
  calc_add/1(out) -> convert_addr/1
  convert_addr/1 -> roachf_2048ch_2GPU_10gbetxsnap_bram_lsb_addr/1
  convert_din1/1 -> roachf_2048ch_2GPU_10gbetxsnap_bram_lsb_data_in/1
  convert_din/1 -> munge_in/1(din)
